simulink model "Lab1_parameter_estimation_student"  (R2025a)
settings: Solver=FixedStepAuto  StartTime=0.0  StopTime=inf  FixedStep=0.001  RelTol=1e-3
values from neighbouring files (symbols this model uses):
  Chirmp_Time = 20    [matlab.mat]
  Mode = 1    [matlab.mat]
  motor_B = 1.02E-04    (= 0.000102)    [Generate_Predict_Graph.m]    (also in Lab1_motor_params_student.m = 8.54e-06; Lab_1_parameter_generate.m = 3.9e-06; Loop_throught_sim.m = 0.0001097471783; Parameter_Estimator.m = 5.51e-05)
  motor_Eff = 0.9997684157    [Generate_Predict_Graph.m]    (also in Lab1_motor_params_student.m = 0.92042; Lab_1_parameter_generate.m = 0.8279549717; Loop_throught_sim.m = 0.9994969307; Parameter_Estimator.m = 0.9997649845)
  motor_J = 0.0002886642529    [Generate_Predict_Graph.m]    (also in Lab1_motor_params_student.m = 0.00015666768297; Lab_1_parameter_generate.m = 0.05438258655; Loop_throught_sim.m = 1.13e-05; Parameter_Estimator.m = 1.27e-05)
  motor_Ke = 0.0439752384    [Generate_Predict_Graph.m]    (also in Lab1_motor_params_student.m = 0.05438258655; Lab_1_parameter_generate.m = 6382.937317; Loop_throught_sim.m = 0.04336937833; Parameter_Estimator.m = 0.04964871404)
  motor_L = 0.02587    [Lab1_motor_params_student.m]    (also in Lab_1_parameter_generate.m = 0.002587; Parameter_Estimator.m = moter_L; Simulation_Parameter_Estimator_Cross_Validation.m = 0.002587)
  motor_R = 3.341    [Lab1_motor_params_student.m]    (also in Lab_1_parameter_generate.m; Simulation_Parameter_Estimator_Cross_Validation.m; matlab.mat = 3.376)
  Ramp_Slope = 0    [matlab.mat]
  Sine_Freq = 0    [matlab.mat]
  Stair_Wait = 0    [matlab.mat]
  Step_Value = 1    [matlab.mat]
libraries: simulink x2
settings Model: PacingRate=5  Creator=tanawatp  LastModifiedBy=ACER
settings DataIOCC: OutputOption=AdditionalOutputTimes  OutputTimes=SDO_OutputTimes  ReturnWorkspaceOutputsName=SDOSimTest_Log
settings RTWCC: GPUComputeCapability=3.5

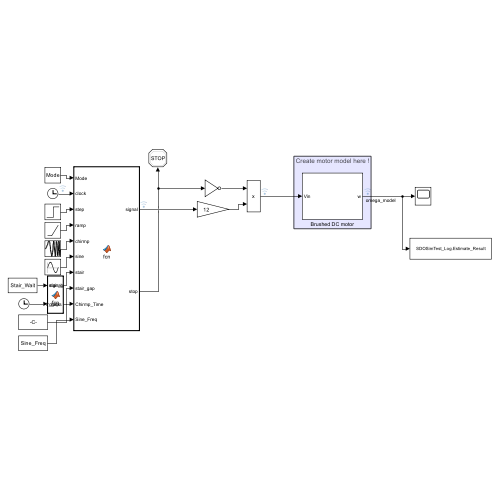
[thumbnail: Simulink's stored preview of the top-level diagram]
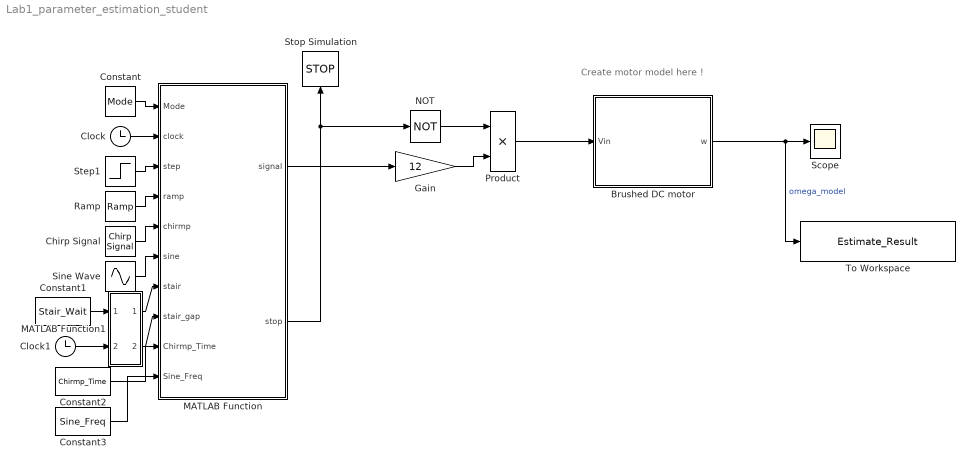
== system Lab1_parameter_estimation_student ==
  note: Create motor model here !
  Brushed DC motor : Subsystem
  Chirp Signal : simulink/Sources/Chirp Signal  f1=0  T=Chirmp_Time  f2=Chirmp_Freq
  Clock : Clock
  Clock1 : Clock
  Constant : Constant  Value=Mode
  Constant1 : Constant  Value=Stair_Wait
  Constant2 : Constant  Value=Chirmp_Time
  Constant3 : Constant  Value=Sine_Freq
  Gain : Gain  Gain=12
  MATLAB Function : MATLAB Function  TreatAsAtomicUnit=on
  MATLAB Function1 : MATLAB Function  TreatAsAtomicUnit=on
  NOT : Logic  Operator=NOT  IconShape=distinctive  AllPortsSameDT=off  OutDataTypeStr=boolean
  Product : Product
  Ramp : simulink/Sources/Ramp  slope=Ramp_Slope  start=0.5  InitialOutput=0
  Scope : Scope
      settings: ActiveDisplayYMinimum=-378.47030938334603  ActiveDisplayYMaximum=349.9210685469078
  Sine Wave : Sin  Frequency=Sine_Freq  Phase=-Sine_Freq/2  SampleTime=0
  Step1 : Step  Time=0.5  After=Step_Value  SampleTime=0
  Stop Simulation : Stop
  To Workspace : ToWorkspace  VariableName=Estimate_Result  SaveFormat=Structure With Time  SampleTime=-1
  wires:
  Brushed DC motor/1(w) -> To Workspace/1, Scope/1  "omega_model"
  Constant3/1 -> MATLAB Function/10(Sine_Freq)
  Product/1 -> Brushed DC motor/1(Vin)
  Constant2/1 -> MATLAB Function/9(Chirmp_Time)
  NOT/1 -> Product/1
  Constant1/1 -> MATLAB Function1/1(stair_gap)
  Step1/1 -> MATLAB Function/3(step)
  MATLAB Function1/2(stair_gaps) -> MATLAB Function/8(stair_gap)
  Clock1/1 -> MATLAB Function1/2(clock)
  Clock/1 -> MATLAB Function/2(clock)
  Gain/1 -> Product/2
  Constant/1 -> MATLAB Function/1(Mode)
  Ramp/1 -> MATLAB Function/4(ramp)
  MATLAB Function/1(signal) -> Gain/1
  Sine Wave/1 -> MATLAB Function/6(sine)
  MATLAB Function1/1(signal) -> MATLAB Function/7(stair)
  MATLAB Function/2(stop) -> NOT/1, Stop Simulation/1
  Chirp Signal/1 -> MATLAB Function/5(chirmp)

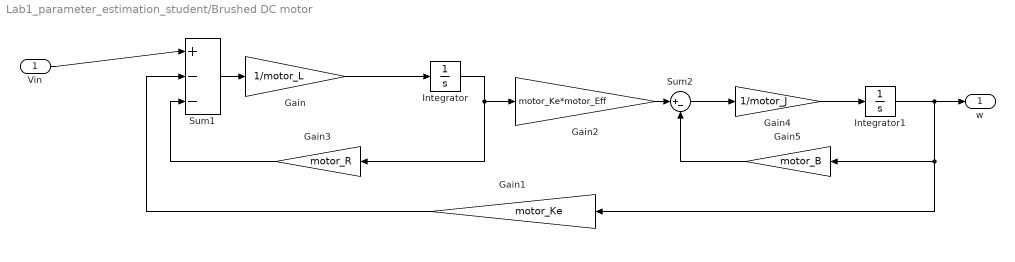
== system Lab1_parameter_estimation_student/Brushed DC motor ==
  Vin : Inport
  Gain : Gain  Gain=1/motor_L
  Gain1 : Gain  Gain=motor_Ke
  Gain2 : Gain  Gain=motor_Ke*motor_Eff
  Gain3 : Gain  Gain=motor_R
  Gain4 : Gain  Gain=1/motor_J
  Gain5 : Gain  Gain=motor_B
  Integrator : Integrator
  Integrator1 : Integrator
  Sum1 : Sum  Inputs=|+--
  Sum2 : Sum  Inputs=|+-
  w : Outport
  wires:
  Vin/1 -> Sum1/1
  Sum1/1 -> Gain/1
  Integrator/1 -> Gain3/1, Gain2/1
  Gain3/1 -> Sum1/3
  Sum2/1 -> Gain4/1
  Gain2/1 -> Sum2/1
  Integrator1/1 -> Gain1/1, Gain5/1, w/1
  Gain5/1 -> Sum2/2
  Gain1/1 -> Sum1/2
  Gain4/1 -> Integrator1/1
  Gain/1 -> Integrator/1

== matlab function Lab1_parameter_estimation_student/MATLAB Function1 ==
  data: signal output; stair_gaps output; stair_gap input; clock input
function [signal,stair_gaps]= fcn(stair_gap,clock)
time_offset = 0.5;
All_signal = 0.25:0.25:1;
clock_usage = clock - time_offset;
if clock_usage < 0
    clock_usage = 0;
end
phase = fix(clock_usage/stair_gap/2);
stair_gaps = stair_gap;
if clock < 0.5
    signal = 0;
    return;
end

if phase <= 3
    buffer = clock_usage - 2*stair_gap*phase;
    if buffer < stair_gap
        signal = All_signal(phase+1);
    else
        signal = 0;
    end
else
    signal = 0;
end

    end

== matlab function Lab1_parameter_estimation_student/MATLAB Function ==
  data: Mode input; signal output; clock input; step input; ramp input; chirmp input; sine input; stair input; stop output; stair_gap input; Chirmp_Time input; Sine_Freq input
function [signal, stop] = fcn(Mode, clock, step, ramp, chirmp, sine, stair, stair_gap, Chirmp_Time,Sine_Freq)

% Default outputs
signal = 0;
stop   = 0;

% Initial 0.5 sec zero output
if clock < 0.5
    return;
end

switch Mode

    case 1   % STEP
        signal = step;
        if clock >= 10.5
            stop = 1;
        end

    case 2   % RAMP
        signal = ramp;
        if signal >= 1
            stop = 1;
        end

    case 3   % CHIRP
        signal = chirmp;
        if clock >= Chirmp_Time
            stop = 1;
        end

    case 4   % SINE
        signal = sine;
        if clock >= 2*pi/Sine_Freq*10
            stop = 1;
        end

  case 5   % STAIR
        signal = stair;

        % 10 amplitudes × (ON + OFF) × stair_gap + 0.5 sec initial
        total_time = 0.5 + 8 * stair_gap;

        if clock >= total_time
            stop = 1;
        end

    otherwise
        signal = 0;
        stop   = 0;
end

end
